simulink model "driveline_dynamics"  (R2021a)
settings: Solver=VariableStepAuto  StartTime=0.0  StopTime=10.0  RelTol=1e-3
values from neighbouring files (symbols this model uses):
  Ie = 0.1782    [main.m]    (also in perc_neg_forces.m)
  Iw = 1000    [main.m]    (also in perc_neg_forces.m)
  R = 0.5    [main.m]    (also in perc_neg_forces.m)
  reff = ( asin(acos(rstat/rw)) / acos(rstat/rw)) * rw    [main.m]    (also in perc_neg_forces.m)
libraries: simulink x2
settings Model: Creator=joaofonseca  LastModifiedBy=joaofonseca

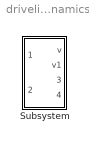
== system driveline_dynamics ==
  Subsystem : Subsystem

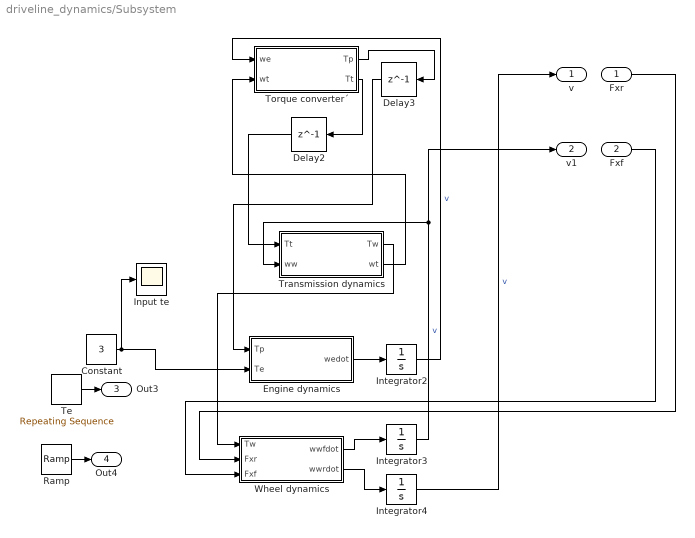
== system driveline_dynamics/Subsystem ==
  Fxr : Inport
  Fxf : Inport  Port=2
  Constant : Constant  Value=3
  Delay2 : Delay  DelayLength=1  InitialCondition=0
  Delay3 : Delay  DelayLength=1  InitialCondition=0
  Engine dynamics : Subsystem
  Input te : Scope
  Integrator2 : Integrator
  Integrator3 : Integrator
  Integrator4 : Integrator
  Ramp : simulink/Sources/Ramp  slope=5  start=2  InitialOutput=2
  Te : simulink/Sources/Repeating Sequence  rep_seq_t=[0 2]  rep_seq_y=[0 10]
  Torque converter´ : Subsystem
  Transmission dynamics : Subsystem
  Wheel dynamics : Subsystem
  v : Outport
  v1 : Outport  Port=2
  Out3 : Outport  Port=3
  Out4 : Outport  Port=4
  wires:
  Ramp/1 -> Out4/1
  Integrator4/1 -> v/1  "v"
  Torque converter´/1(Tp) -> Delay3/1
  Constant/1 -> Input te/1, Engine dynamics/2(Te)
  Integrator3/1 -> v1/1, Transmission dynamics/2(ww)  "v"
  Integrator2/1 -> Torque converter´/1(we)  "v"
  Transmission dynamics/1(Tw) -> Wheel dynamics/1(Tw)
  Engine dynamics/1(wedot) -> Integrator2/1
  Fxr/1 -> Wheel dynamics/2(Fxr)
  Wheel dynamics/2(wwrdot) -> Integrator4/1
  Delay2/1 -> Transmission dynamics/1(Tt)
  Fxf/1 -> Wheel dynamics/3(Fxf)
  Te/1 -> Out3/1
  Delay3/1 -> Engine dynamics/1(Tp)
  Transmission dynamics/2(wt) -> Torque converter´/2(wt)
  Torque converter´/2(Tt) -> Delay2/1
  Wheel dynamics/1(wwfdot) -> Integrator3/1

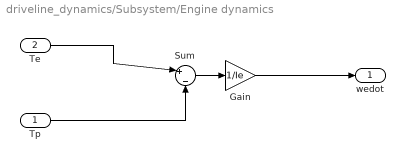
== system driveline_dynamics/Subsystem/Engine dynamics ==
  Tp : Inport
  Te : Inport  Port=2
  Gain : Gain  Gain=1/Ie
  Sum : Sum  Inputs=|+|-
  wedot : Outport
  wires:
  Te/1 -> Sum/1
  Tp/1 -> Sum/2
  Sum/1 -> Gain/1
  Gain/1 -> wedot/1

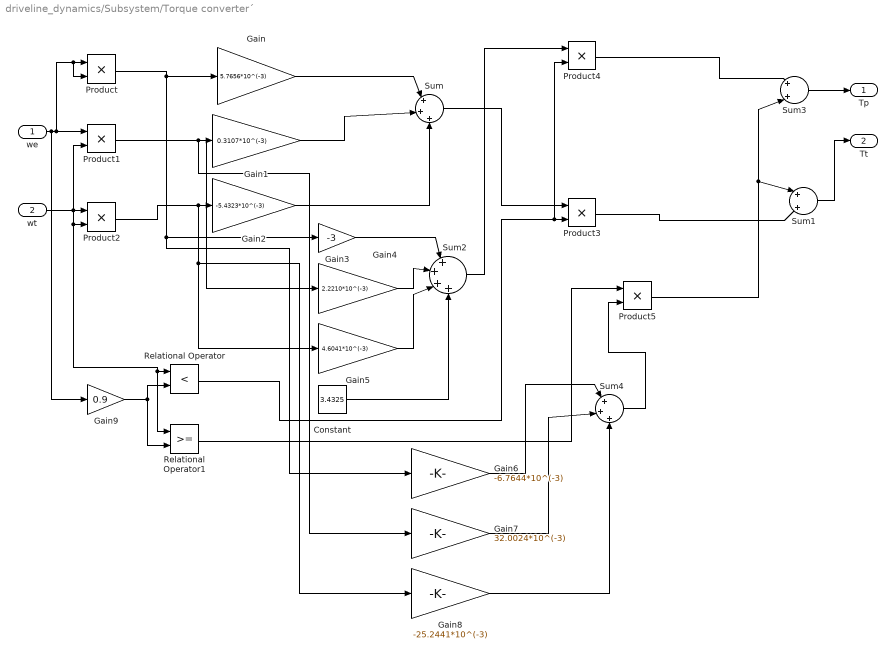
== system driveline_dynamics/Subsystem/Torque converter´ ==
  we : Inport
  wt : Inport  Port=2
  Constant : Constant  Value=3.4325
  Gain : Gain  Gain=5.7656*10^(-3)
  Gain1 : Gain  Gain=0.3107*10^(-3)
  Gain2 : Gain  Gain=-5.4323*10^(-3)
  Gain3 : Gain  Gain=-3
  Gain4 : Gain  Gain=2.2210*10^(-3)
  Gain5 : Gain  Gain=4.6041*10^(-3)
  Gain6 : Gain  Gain=-6.7644*10^(-3)
  Gain7 : Gain  Gain=32.0024*10^(-3)
  Gain8 : Gain  Gain=-25.2441*10^(-3)
  Gain9 : Gain  Gain=0.9
  Product{,1..5} (6 alike) : Product
  Relational Operator : RelationalOperator  Operator=<  OutDataTypeStr=boolean  ZeroCross=off  RndMeth=Simplest
  Relational Operator1 : RelationalOperator  OutDataTypeStr=boolean  ZeroCross=off  RndMeth=Simplest
  Sum : Sum  Inputs=|+|+|+
  Sum1 : Sum  Inputs=|+|+|
  Sum2 : Sum  Inputs=|+|+|+|+
  Sum3 : Sum  Inputs=|+|+|
  Sum4 : Sum  Inputs=|+|+|+
  Tp : Outport
  Tt : Outport  Port=2
  wires:
  wt/1 -> Product2/2, Relational Operator1/1, Relational Operator/1, Product2/1, Product1/2
  we/1 -> Product1/1, Product/2, Product/1, Gain9/1
  Product/1 -> Gain3/1, Gain6/1, Gain/1
  Product1/1 -> Gain4/1, Gain1/1, Gain7/1
  Product2/1 -> Gain5/1, Gain8/1, Gain2/1
  Gain/1 -> Sum/1
  Gain1/1 -> Sum/2
  Gain2/1 -> Sum/3
  Relational Operator/1 -> Product4/2, Product3/2
  Sum/1 -> Product3/1
  Product3/1 -> Sum1/2
  Sum1/1 -> Tt/1
  Constant/1 -> Sum2/4
  Gain5/1 -> Sum2/3
  Gain4/1 -> Sum2/2
  Gain3/1 -> Sum2/1
  Sum3/1 -> Tp/1
  Product4/1 -> Sum3/1
  Sum2/1 -> Product4/1
  Gain8/1 -> Sum4/3
  Gain7/1 -> Sum4/2
  Gain6/1 -> Sum4/1
  Relational Operator1/1 -> Product5/1
  Sum4/1 -> Product5/2
  Product5/1 -> Sum1/1, Sum3/2
  Gain9/1 -> Relational Operator1/2, Relational Operator/2

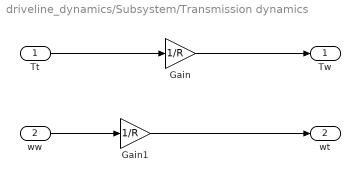
== system driveline_dynamics/Subsystem/Transmission dynamics ==
  Tt : Inport
  ww : Inport  Port=2
  Gain : Gain  Gain=1/R
  Gain1 : Gain  Gain=1/R
  Tw : Outport
  wt : Outport  Port=2
  wires:
  Tt/1 -> Gain/1
  ww/1 -> Gain1/1
  Gain/1 -> Tw/1
  Gain1/1 -> wt/1

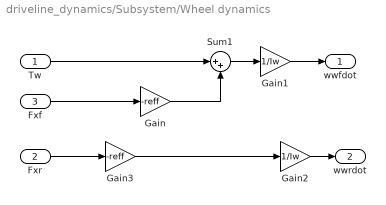
== system driveline_dynamics/Subsystem/Wheel dynamics ==
  Tw : Inport
  Fxr : Inport  Port=2
  Fxf : Inport  Port=3
  Gain : Gain  Gain=-reff
  Gain1 : Gain  Gain=1/Iw
  Gain2 : Gain  Gain=1/Iw
  Gain3 : Gain  Gain=-reff
  Sum1 : Sum  Inputs=|++
  wwfdot : Outport
  wwrdot : Outport  Port=2
  wires:
  Tw/1 -> Sum1/1
  Gain/1 -> Sum1/2
  Sum1/1 -> Gain1/1
  Gain1/1 -> wwfdot/1
  Gain2/1 -> wwrdot/1
  Fxf/1 -> Gain/1
  Fxr/1 -> Gain3/1
  Gain3/1 -> Gain2/1
